simulink model "hc12_led"  (Simulink 6.0)
settings: Solver=FixedStepDiscrete  StartTime=0.0  StopTime=50.0  FixedStep=hc12_base_st  RelTol=1e-3
PreLoadFcn:
  | [hc12_base_st] = hc12_closest_st(0.065536,16000000);
undefined symbols (not defined in the file or in its folder): hc12_base_st
libraries: simulink x2, hc12drivers x2
settings Model: Creator=The MathWorks Inc.  LastModifiedBy=batserve  ExtModeAutoUpdateStatusClock=off  ProdHWDeviceType=Motorola HC12
settings DataIOCC: SignalLoggingName=sigsOut
settings OptimizationCC: InlineParams=on  InlineInvariantSignals=off  ZeroExternalMemoryAtStartup=off  ZeroInternalMemoryAtStartup=off  OptimizeModelRefInitCode=on  LifeSpan=1
settings DebuggingCC: CheckExecutionContextPreStartOutputMsg=on  CheckExecutionContextRuntimeOutputMsg=on  SolverPrmCheckMsg=none  ParameterPrecisionLossMsg=none  UnnecessaryDatatypeConvMsg=warning
settings HardwareCC: ProdBitPerInt=16  ProdEndianess=BigEndian  ProdWordSize=16  ProdHWDeviceType=Motorola HC12
settings RTWCC: SystemTargetFile=hc12.tlc  TemplateMakefile=hc12_default_tmf  GenerateReport=on  ProcessScript=hc12_make_rtw_hook  IncludeHyperlinkInReport=on  LaunchReport=on
settings CodeAppCC: IgnoreCustomStorageClasses=off
settings STFCustomTargetCC: TargetFcnLib=ansi_tfl_tmw.mat  GenFloatMathFcnCalls=ANSI_C  ModelReferenceCompliant=off  IncludeMdlTerminateFcn=off  CombineOutputUpdateFcns=on  SuppressErrorStatus=on  ERTCustomFileBanners=on  SupportAbsoluteTime=off  SupportNonFinite=off  SupportComplex=off  PurelyIntegerCode=on  SupportContinuousTime=off  SupportNonInlinedSFcns=off  SystemTargetFile=hc12.tlc
settings ERTTargetCC: TargetFcnLib=ansi_tfl_tmw.mat  GenFloatMathFcnCalls=ANSI_C  ModelReferenceCompliant=off  IncludeMdlTerminateFcn=off  SuppressErrorStatus=on  SupportAbsoluteTime=off  SupportNonFinite=off  SupportComplex=off  PurelyIntegerCode=on  RootIOFormat=Individual Arguments  ERTCustomFileTemplate=hc12_file_process.tlc  InitialValueSource=Model
settings CustomProperty: DataType=RTWOptions_EnumType__toolbox_rtw_targets_hc12_hc12_hc12_PWMPrescalerA  Value=1
settings EnumStrPairs: String=1

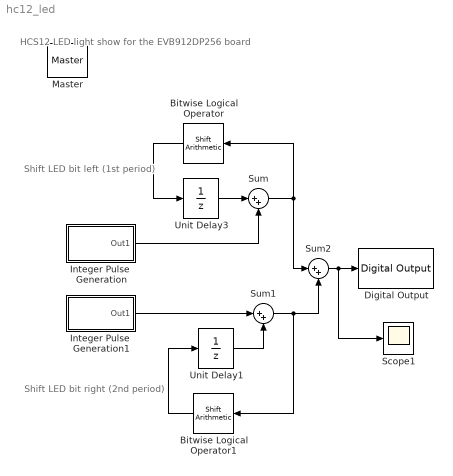
== system hc12_led ==
  note: Shift LED bit left
      | (1st period)
  note: Shift LED bit right
      | (2nd period)
  note: HCS12 LED light show
      | for the EVB912DP256 board
  Bitwise Logical Operator : simulink/Logic and Bit Operations/Shift Arithmetic  Orientation=left  nBitShiftRight=-1  nBinPtShiftRight=0
  Bitwise Logical Operator1 : simulink/Logic and Bit Operations/Shift Arithmetic  Orientation=left  nBitShiftRight=1  nBinPtShiftRight=0
  Digital Output : hc12drivers/Digital Output  doport=B
  Integer Pulse  Generation : Subsystem  PropExecContextAcrossSSBoundary=on
  Integer Pulse  Generation1 : Subsystem  PropExecContextAcrossSSBoundary=on
  Master : hc12drivers/Master  Tag=HardwareResourceMaster  Priority=100  osc=16000000  desiredST=hc12_base_st
  Scope1 : Scope
      settings: TimeRange=5  YMin=0  YMax=300  MaxDataPoints=50000
  Sum : Sum  Inputs=|++  SaturateOnIntegerOverflow=on
  Sum1 : Sum  Inputs=|++  SaturateOnIntegerOverflow=on
  Sum2 : Sum  Inputs=|++  SaturateOnIntegerOverflow=on
  Unit Delay1 : UnitDelay  X0=uint8(0)  SampleTime=hc12_base_st
  Unit Delay3 : UnitDelay  X0=uint8(0)  SampleTime=hc12_base_st
  wires:
  Integer Pulse  Generation/1(Out1) -> Sum/2
  Unit Delay3/1 -> Sum/1
  Sum/1 -> Bitwise Logical Operator/1, Sum2/1
  Bitwise Logical Operator/1 -> Unit Delay3/1
  Bitwise Logical Operator1/1 -> Unit Delay1/1
  Sum2/1 -> Scope1/1, Digital Output/1
  Unit Delay1/1 -> Sum1/2
  Integer Pulse  Generation1/1(Out1) -> Sum1/1
  Sum1/1 -> Sum2/2, Bitwise Logical Operator1/1

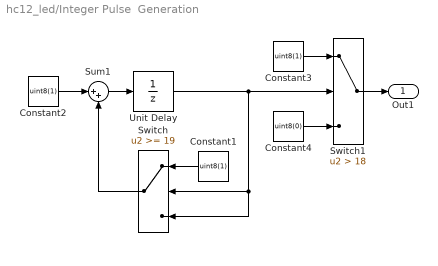
== system hc12_led/Integer Pulse  Generation ==
  Constant1 : Constant  Orientation=left  Value=uint8(1)
  Constant2 : Constant  Value=uint8(1)
  Constant3 : Constant  Value=uint8(1)
  Constant4 : Constant  Value=uint8(0)
  Sum1 : Sum  Inputs=|++  SaturateOnIntegerOverflow=on
  Switch : Switch  Orientation=left  Threshold=19  SaturateOnIntegerOverflow=on  InputSameDT=on
  Switch1 : Switch  Criteria=u2 > Threshold  Threshold=18  SaturateOnIntegerOverflow=on
  Unit Delay : UnitDelay  X0=uint8(0)  SampleTime=hc12_base_st
  Out1 : Outport
  wires:
  Switch1/1 -> Out1/1
  Constant4/1 -> Switch1/3
  Constant3/1 -> Switch1/1
  Switch/1 -> Sum1/2
  Constant2/1 -> Sum1/1
  Sum1/1 -> Unit Delay/1
  Constant1/1 -> Switch/1
  Unit Delay/1 -> Switch/3, Switch/2, Switch1/2

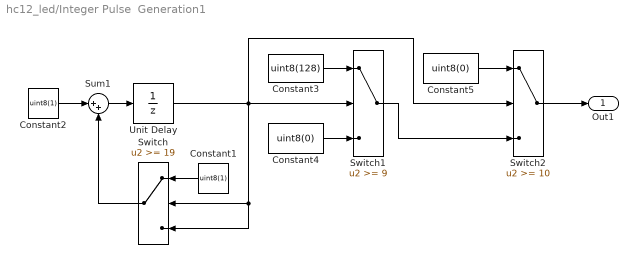
== system hc12_led/Integer Pulse  Generation1 ==
  Constant1 : Constant  Orientation=left  Value=uint8(1)
  Constant2 : Constant  Value=uint8(1)
  Constant3 : Constant  Value=uint8(128)
  Constant4 : Constant  Value=uint8(0)
  Constant5 : Constant  Value=uint8(0)
  Sum1 : Sum  Inputs=|++  SaturateOnIntegerOverflow=on
  Switch : Switch  Orientation=left  Threshold=19  SaturateOnIntegerOverflow=on  InputSameDT=on
  Switch1 : Switch  Threshold=9  SaturateOnIntegerOverflow=on
  Switch2 : Switch  Threshold=10  SaturateOnIntegerOverflow=on
  Unit Delay : UnitDelay  X0=uint8(0)  SampleTime=hc12_base_st
  Out1 : Outport
  wires:
  Constant5/1 -> Switch2/1
  Switch1/1 -> Switch2/3
  Switch2/1 -> Out1/1
  Unit Delay/1 -> Switch2/2, Switch1/2, Switch/2, Switch/3
  Constant1/1 -> Switch/1
  Sum1/1 -> Unit Delay/1
  Constant2/1 -> Sum1/1
  Switch/1 -> Sum1/2
  Constant3/1 -> Switch1/1
  Constant4/1 -> Switch1/3
